simulink model "P4p2_no_integral"  (R2014a)
settings: Solver=ode1  StartTime=0.0  StopTime=inf  FixedStep=0.002  RelTol=1e-3
PostLoadFcn:
  | qc_set_target_type(getConfigSet(bdroot, 'QUARC Default Target Configuration'));
values from neighbouring files (symbols this model uses):
  A_e = [0  1 0 0 0 0 ... (first row only)    [P4p2_no_integral_init.m]
  B_e = [0  0 ... (first row only)    [P4p2_no_integral_init.m]
  C_e = [1 0 0 0 0 0 ... (first row only)    [P4p2_no_integral_init.m]
  L_e = place(A_e', C_e', q).'    [P4p2_no_integral_init.m]
undefined symbols (not defined in the file or in its folder): elevation_offset, HIL, Joystick_gain_x, Joystick_gain_y, K, P, qc_get_step_size, Vs_star_meas
libraries: quarc_library x8, simulink_extras x7
settings Model: SimulationMode=external  ExtModeTrigDuration=5000  Creator=Rchan  LastModifiedBy=rendellc
settings SolverCC: PositivePriorityOrder=on
settings DataIOCC: SignalLoggingSaveFormat=ModelDataLogs
settings OptimizationCC: ExpressionDepthLimit=2147483647  InitFltsAndDblsToZero=on
settings DebuggingCC: SaveWithParameterizedLinksMsg=none  UnderspecifiedInitializationDetection=Classic  MultiTaskDSMMsg=warning  MultiTaskCondExecSysMsg=none  FcnCallInpInsideContextMsg=UseLocalSettings  StateNameClashWarn=warning
settings RTWCC: SystemTargetFile=quarc_win64.tlc  TemplateMakefile=quarc_default_tmf  Description=QUARC Win64 Target  ProcessScript=quarc_win64_make_rtw_hook
settings STFCustomTargetCC: CPPClassGenCompliant=on
settings GRTTargetCC: ParMdlRefBuildCompliant=off  CompOptLevelCompliant=off  CombineOutputUpdateFcns=off  MatFileLogging=off  GRTInterface=on  ExtMode=on  ExtModeMexFile=quarc_comm

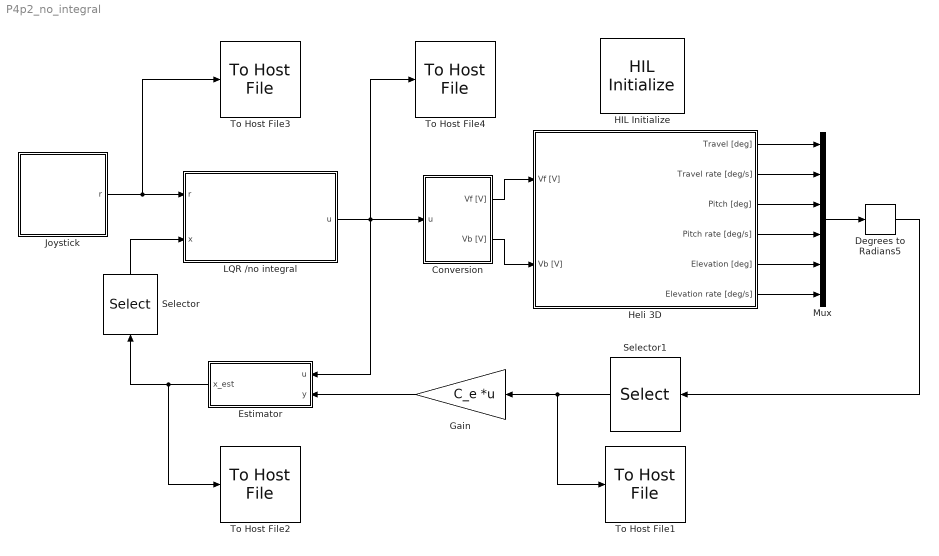
== system P4p2_no_integral ==
  "Conversion " : Subsystem
  Degrees to Radians5 : simulink_extras/Transformations/Degrees to Radians
  Estimator : Subsystem
  Gain : Gain  Gain=C_e  Multiplication=Matrix(K*u) (u vector)
  HIL Initialize : quarc_library/Data Acquisition/Generic/Configuration/HIL Initialize  Priority=-99  object_name=HIL-1  board_type=q8_usb  board_number=0  board_options=update_rate=normal;decimation=1  exclusive=off  active=off  hardware_clocks=[0:2]  clock_modes=[]  initial_clock_frequencies=[]  set_clock_params_at_start=off  set_clock_params_at_switch_in=off  set_clock_frequencies_at_start=off  set_clock_frequencies_at_switch_in=off  analog_input_channels=[0:7]  analog_input_maximums=10  analog_input_minimums=-10  set_analog_input_params_at_start=on  set_analog_input_params_at_switch_in=off  analog_output_channels=[0:7]  analog_output_maximums=10  analog_output_minimums=-10  initial_analog_outputs=[0]  final_analog_outputs=[0]  watchdog_analog_outputs=0  set_analog_output_params_at_start=on  set_analog_output_params_at_switch_in=off  set_analog_outputs_at_start=on  set_analog_outputs_at_switch_in=off  set_analog_outputs_at_terminate=on  set_analog_outputs_at_switch_out=off  set_analog_outputs_on_watchdog=off  digital_input_channels=[]  digital_output_channels=[]  digital_output_configuration=[]  initial_digital_outputs=[1]  final_digital_outputs=[1]  watchdog_digital_outputs=[1]  set_digital_output_params_at_start=off  set_digital_output_params_at_switch_in=off  set_digital_outputs_at_start=on  set_digital_outputs_at_switch_in=off  set_digital_outputs_at_terminate=on  set_digital_outputs_at_switch_out=off  set_digital_outputs_on_watchdog=off  encoder_channels=[0:7]  quadrature=[4]  encoder_filter_frequency=[]  initial_encoder_counts=[0]  set_encoder_params_at_start=on  set_encoder_params_at_switch_in=off  set_encoder_counts_at_start=on  set_encoder_counts_at_switch_in=off  pwm_channels=[0:7]  pwm_modes=0  pwm_frequency=99.532799999999995e6/4095  pwm_configuration=[0]  pwm_alignment=[0]  pwm_polarity=[1]  pwm_leading_deadband=[0]  pwm_trailing_deadband=[0]  initial_pwm_outputs=[0]  final_pwm_outputs=[0]  watchdog_pwm_outputs=[0]  set_pwm_params_at_start=on  set_pwm_params_at_switch_in=off  set_pwm_outputs_at_start=on  set_pwm_outputs_at_switch_in=off  set_pwm_outputs_at_terminate=on  set_pwm_outputs_at_switch_out=off  set_pwm_outputs_on_watchdog=off  other_output_channels=[]  initial_other_outputs=[]  final_other_outputs=[]  watchdog_other_outputs=[]  set_other_outputs_at_start=off  set_other_outputs_at_switch_in=off  set_other_outputs_at_terminate=off  set_other_outputs_at_switch_out=off  set_other_outputs_on_watchdog=off
  Heli 3D : Subsystem
  Joystick : Subsystem
      mask Display: image('../Common/joy_img.png');
  LQR /no integral : Subsystem
  Mux : Mux  Inputs=6
  Selector : Selector  InputPortWidth=6  Indices=[1 2 4]
  Selector1 : Selector  InputPortWidth=6  Indices=[3 4 5 6 1 2]
  To Host File1 : quarc_library/Sinks/To Host/To Host File  file_name=..\..\data\Part 4\%m_x.mat  variable_name=x  decimation=1  sample_time=-1  file_format=MAT-file v.4  options=No header or footer  append=off  final_file_name=..\..\data\Part 4\P4p2_no_integral_x.mat
  To Host File2 : quarc_library/Sinks/To Host/To Host File  file_name=..\..\data\Part 4\%m_x_est.mat  variable_name=x_est  decimation=1  sample_time=-1  file_format=MAT-file v.4  options=No header or footer  append=off  final_file_name=..\..\data\Part 4\P4p2_no_integral_x_est.mat
  To Host File3 : quarc_library/Sinks/To Host/To Host File  file_name=..\..\data\Part 4\%m_ref.mat  variable_name=ref  decimation=1  sample_time=-1  file_format=MAT-file v.4  options=No header or footer  append=off  final_file_name=..\..\data\Part 4\P4p2_no_integral_ref.mat
  To Host File4 : quarc_library/Sinks/To Host/To Host File  file_name=..\..\data\Part 4\%m_u.mat  variable_name=u  decimation=1  sample_time=-1  file_format=MAT-file v.4  options=No header or footer  append=off  final_file_name=..\..\data\Part 4\P4p2_no_integral_u.mat
  wires:
  "Conversion "/2(Vb [V]) -> Heli 3D/2(Vb [V])
  "Conversion "/1(Vf [V]) -> Heli 3D/1(Vf [V])
  Heli 3D/1(Travel [deg]) -> Mux/1
  Heli 3D/2(Travel rate [deg/s]) -> Mux/2
  Heli 3D/3(Pitch [deg]) -> Mux/3
  Heli 3D/4(Pitch rate [deg/s]) -> Mux/4
  Heli 3D/6(Elevation rate [deg/s]) -> Mux/6
  Heli 3D/5(Elevation [deg]) -> Mux/5
  Mux/1 -> Degrees to Radians5/1
  Estimator/1(x_est) -> To Host File2/1, Selector/1
  Selector/1 -> LQR /no integral/2(x)
  Degrees to Radians5/1 -> Selector1/1
  Selector1/1 -> To Host File1/1, Gain/1
  Gain/1 -> Estimator/2(y)
  LQR /no integral/1(u) -> To Host File4/1, Estimator/1(u), "Conversion "/1(u)
  Joystick/1(r) -> To Host File3/1, LQR /no integral/1(r)

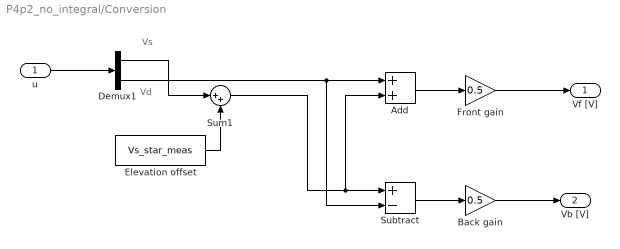
== system P4p2_no_integral/Conversion  ==
  note: Vs
  note: Vd
  u : Inport
  Add : Sum
  Back gain : Gain  Gain=0.5
  Demux1 : Demux  Outputs=2
  Elevation offset : Constant  Value=Vs_star_meas
  Front gain : Gain  Gain=0.5
  Subtract : Sum  Inputs=+-
  Sum1 : Sum  Inputs=|++
  Vf [V] : Outport
  Vb [V] : Outport  Port=2
  wires:
  Subtract/1 -> Back gain/1
  Back gain/1 -> Vb [V]/1
  Add/1 -> Front gain/1
  Front gain/1 -> Vf [V]/1
  u/1 -> Demux1/1
  Demux1/2 -> Subtract/2, Add/1
  Demux1/1 -> Sum1/1
  Sum1/1 -> Add/2, Subtract/1
  Elevation offset/1 -> Sum1/2

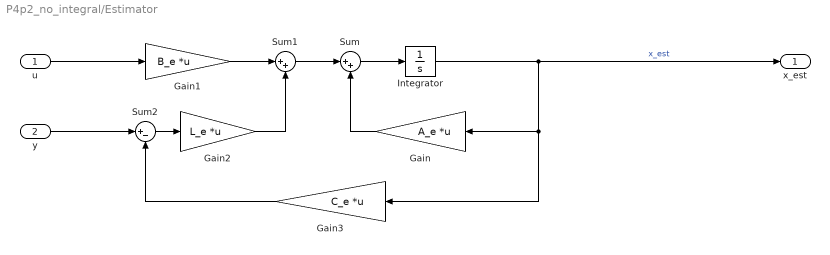
== system P4p2_no_integral/Estimator ==
  u : Inport
  y : Inport  Port=2
  Gain : Gain  Gain=A_e  Multiplication=Matrix(K*u) (u vector)
  Gain1 : Gain  Gain=B_e  Multiplication=Matrix(K*u) (u vector)
  Gain2 : Gain  Gain=L_e  Multiplication=Matrix(K*u) (u vector)
  Gain3 : Gain  Gain=C_e  Multiplication=Matrix(K*u) (u vector)
  Integrator : Integrator
  Sum : Sum  Inputs=|++
  Sum1 : Sum  Inputs=|++
  Sum2 : Sum  Inputs=|+-
  x_est : Outport
  wires:
  u/1 -> Gain1/1
  Sum/1 -> Integrator/1
  Integrator/1 -> Gain3/1, Gain/1, x_est/1  "x_est"
  Gain/1 -> Sum/2
  Sum1/1 -> Sum/1
  Gain1/1 -> Sum1/1
  Gain2/1 -> Sum1/2
  y/1 -> Sum2/1
  Sum2/1 -> Gain2/1
  Gain3/1 -> Sum2/2

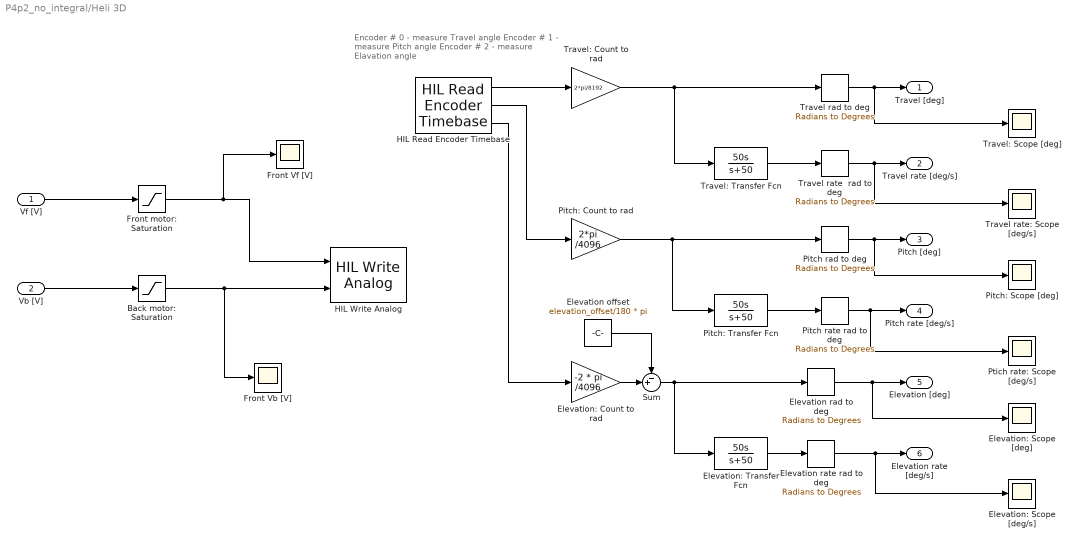
== system P4p2_no_integral/Heli 3D ==
  note: Encoder # 0 - measure Travel angle
      | Encoder # 1 - measure Pitch angle
      | Encoder # 2 - measure Elavation angle
  Vf [V] : Inport
  Vb [V] : Inport  Port=2
  Back motor: Saturation : Saturate  UpperLimit=5  LowerLimit=-5
  Elevation offset : Constant  Value=elevation_offset/180 * pi
  Elevation rad to deg : simulink_extras/Transformations/Radians to Degrees
  Elevation rate rad to deg : simulink_extras/Transformations/Radians to Degrees
  Elevation: Count to rad : Gain  Gain=-2 * pi /4096
  Elevation: Scope [deg/s] : Scope
      settings: YMin=-1500  YMax=250  SaveName=ScopeData13
  Elevation: Scope [deg] : Scope
      settings: YMax=45  SaveName=ScopeData12
  Elevation: Transfer Fcn : TransferFcn  Numerator=[50 0]  Denominator=[1 50]
  Front Vb [V] : Scope
      settings: YMin=-2  SaveName=ScopeData2
  Front Vf [V] : Scope
      settings: YMin=-2
  Front motor: Saturation : Saturate  UpperLimit=5  LowerLimit=-5
  HIL Read Encoder Timebase : quarc_library/Data Acquisition/Generic/Timebases/HIL Read Encoder Timebase  object_name=HIL-1  clock=0  channels=[0:2]  samples_in_buffer=max(ceil(1/qc_get_step_size), 1)  active=on  vector_output=off  data_type_mode=Inherit via back propagation  data_type=double
  HIL Write Analog : quarc_library/Data Acquisition/Generic/Immediate I//O/HIL Write Analog  object_name=HIL-1  channels=[0:1]  sample_time=-1  active=off  vector_input=off
  Pitch rad to deg : simulink_extras/Transformations/Radians to Degrees
  Pitch rate rad to deg : simulink_extras/Transformations/Radians to Degrees
  Pitch: Count to rad : Gain  Gain=2*pi /4096
  Pitch: Scope [deg] : Scope
      settings: YMin=-80  YMax=80  SaveName=ScopeData10
  Pitch: Transfer Fcn : TransferFcn  Numerator=[50 0]  Denominator=[1 50]
  Ptich rate: Scope [deg/s] : Scope
      settings: YMin=-25  YMax=35  SaveName=ScopeData11
  Sum : Sum  Inputs=-+|
  Travel rad to deg : simulink_extras/Transformations/Radians to Degrees
  Travel rate  rad to deg : simulink_extras/Transformations/Radians to Degrees
  Travel rate: Scope [deg/s] : Scope
      settings: YMin=-30  YMax=70  SaveName=ScopeData9
  Travel: Count to rad : Gain  Gain=2*pi/8192
  Travel: Scope [deg] : Scope
      settings: YMin=-250  YMax=2250  SaveName=ScopeData8
  Travel: Transfer Fcn : TransferFcn  Numerator=[50 0]  Denominator=[1 50]
  Travel [deg] : Outport
  Travel rate [deg/s] : Outport  Port=2
  Pitch [deg] : Outport  Port=3
  Pitch rate [deg/s] : Outport  Port=4
  Elevation [deg] : Outport  Port=5
  Elevation rate [deg/s] : Outport  Port=6
  wires:
  HIL Read Encoder Timebase/1 -> Travel: Count to rad/1
  HIL Read Encoder Timebase/2 -> Pitch: Count to rad/1
  HIL Read Encoder Timebase/3 -> Elevation: Count to rad/1
  Travel: Count to rad/1 -> Travel: Transfer Fcn/1, Travel rad to deg/1
  Travel: Transfer Fcn/1 -> Travel rate  rad to deg/1
  Pitch: Count to rad/1 -> Pitch: Transfer Fcn/1, Pitch rad to deg/1
  Pitch: Transfer Fcn/1 -> Pitch rate rad to deg/1
  Elevation: Transfer Fcn/1 -> Elevation rate rad to deg/1
  Travel rad to deg/1 -> Travel: Scope [deg]/1, Travel [deg]/1
  Travel rate  rad to deg/1 -> Travel rate: Scope [deg/s]/1, Travel rate [deg/s]/1
  Pitch rad to deg/1 -> Pitch: Scope [deg]/1, Pitch [deg]/1
  Pitch rate rad to deg/1 -> Ptich rate: Scope [deg/s]/1, Pitch rate [deg/s]/1
  Elevation rad to deg/1 -> Elevation: Scope [deg]/1, Elevation [deg]/1
  Elevation rate rad to deg/1 -> Elevation: Scope [deg/s]/1, Elevation rate [deg/s]/1
  Vf [V]/1 -> Front motor: Saturation/1
  Vb [V]/1 -> Back motor: Saturation/1
  Back motor: Saturation/1 -> Front Vb [V]/1, HIL Write Analog/2
  Elevation: Count to rad/1 -> Sum/2
  Sum/1 -> Elevation: Transfer Fcn/1, Elevation rad to deg/1
  Elevation offset/1 -> Sum/1
  Front motor: Saturation/1 -> Front Vf [V]/1, HIL Write Analog/1

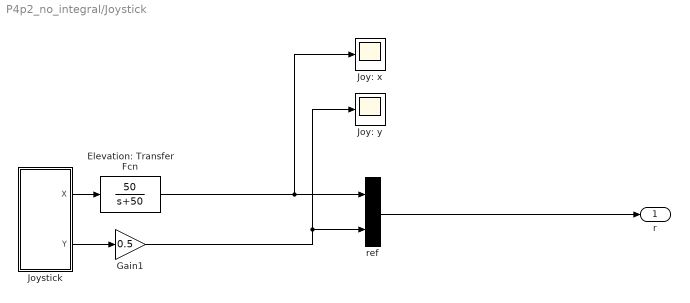
== system P4p2_no_integral/Joystick ==
  Elevation: Transfer Fcn : TransferFcn  Numerator=[0 50]  Denominator=[1 50]
  Gain1 : Gain  Gain=0.5
  Joy: x : Scope
  Joy: y : Scope
      settings: SaveName=ScopeData3
  Joystick : Subsystem
  ref : Concatenate
  r : Outport
  wires:
  Elevation: Transfer Fcn/1 -> Joy: x/1, ref/1
  Joystick/2(Y) -> Gain1/1
  ref/1 -> r/1
  Gain1/1 -> Joy: y/1, ref/2
  Joystick/1(X) -> Elevation: Transfer Fcn/1

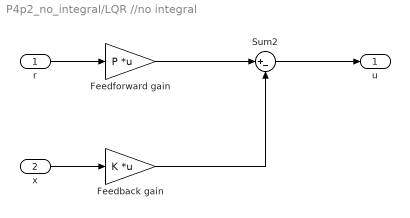
== system P4p2_no_integral/LQR //no integral ==
  r : Inport
  x : Inport  Port=2
  Feedback gain : Gain  Gain=K  Multiplication=Matrix(K*u)
  Feedforward gain : Gain  Gain=P  Multiplication=Matrix(K*u)
  Sum2 : Sum  Inputs=|+-
  u : Outport
  wires:
  x/1 -> Feedback gain/1
  Feedforward gain/1 -> Sum2/1
  Feedback gain/1 -> Sum2/2
  Sum2/1 -> u/1
  r/1 -> Feedforward gain/1

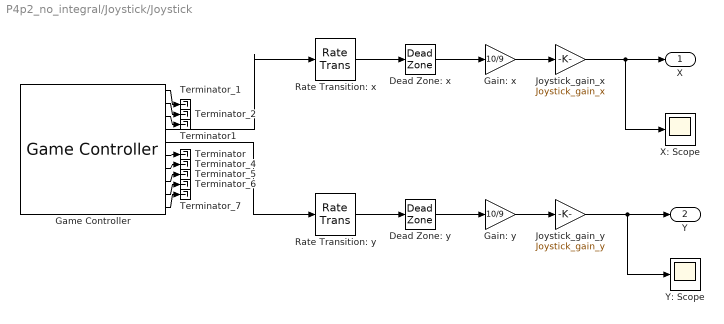
== system P4p2_no_integral/Joystick/Joystick ==
  Dead Zone: x : DeadZone  LowerValue=-0.1  UpperValue=0.1  SaturateOnIntegerOverflow=on
  Dead Zone: y : DeadZone  LowerValue=-0.1  UpperValue=0.1  SaturateOnIntegerOverflow=on
  Gain: x : Gain  Gain=10/9
  Gain: y : Gain  Gain=10/9
  Game Controller : quarc_library/Devices/Peripherals/Target/Game Controller  controller=1  buffer_size=12  deadzone=[]  saturation=[]  sample_time=max(qc_get_step_size, 0.01)  auto_center=off  enabled=on
  Joystick_gain_x : Gain  Gain=Joystick_gain_x
  Joystick_gain_y : Gain  Gain=Joystick_gain_y
  Rate Transition: x : RateTransition
  Rate Transition: y : RateTransition
  Terminator : Terminator
  Terminator1 : Terminator
  Terminator_{1..2,4..7} (6 alike) : Terminator
  X: Scope : Scope
      settings: YMin=-1  YMax=1  SaveName=ScopeData7
  Y: Scope : Scope
      settings: YMin=-10  YMax=10  SaveName=ScopeData5
  X : Outport
  Y : Outport  Port=2
  wires:
  Rate Transition: y/1 -> Dead Zone: y/1
  Rate Transition: x/1 -> Dead Zone: x/1
  Game Controller/5 -> Rate Transition: y/1
  Game Controller/4 -> Rate Transition: x/1
  Game Controller/1 -> Terminator_1/1
  Game Controller/2 -> Terminator_2/1
  Game Controller/7 -> Terminator_4/1
  Game Controller/8 -> Terminator_5/1
  Game Controller/9 -> Terminator_6/1
  Game Controller/10 -> Terminator_7/1
  Game Controller/3 -> Terminator1/1
  Game Controller/6 -> Terminator/1
  Dead Zone: x/1 -> Gain: x/1
  Dead Zone: y/1 -> Gain: y/1
  Gain: x/1 -> Joystick_gain_x/1
  Gain: y/1 -> Joystick_gain_y/1
  Joystick_gain_x/1 -> X/1, X: Scope/1
  Joystick_gain_y/1 -> Y: Scope/1, Y/1
